simulink model "state_flow_with_system"  (R2023a)
settings: Solver=ode4  StartTime=0.0  StopTime=35  FixedStep=0.01
settings Model: Creator=Nada Tamer  LastModifiedBy=Dina
settings SolverCC: MaxConsecutiveMinStep=10  ZeroCrossAlgorithm=Adaptive
settings DebuggingCC: TimeAdjustmentMsg=warning  IgnoredZcDiagnostic=none

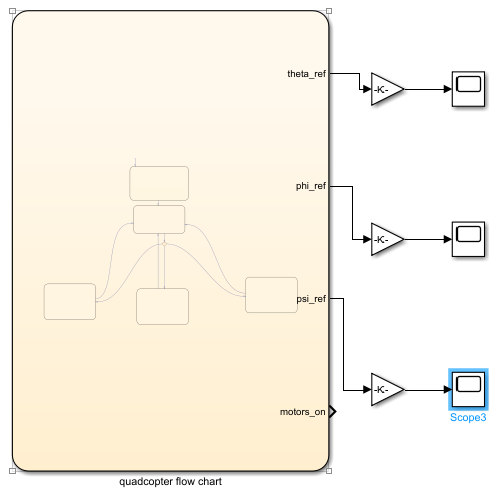
[thumbnail: Simulink's stored preview of the top-level diagram]
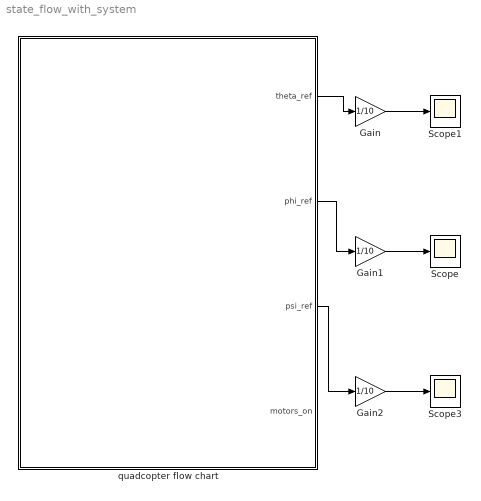
== system state_flow_with_system ==
  Gain : Gain  Gain=1/10
  Gain1 : Gain  Gain=1/10
  Gain2 : Gain  Gain=1/10
  Scope : Scope
  Scope1 : Scope
  Scope3 : Scope
  quadcopter flow chart : Stateflow chart  TreatAsAtomicUnit=on
      settings: PortSchema="{\"entries\":[{\"content\":{\"sides\":[{\"content\":{},\"type\":\"ConnectorPlacement.EquallySpacedRectSide\",\"uuid\":\"56c2e152-afcd-40b1-8237-a18b8b05acf4\"},{\"content\":{\"connectorIds\":[\"Out2\",\"Out1\",\"Out3\",\"Out4\"],\"side\":\"RIGHT\"},\"type\":\"ConnectorPlacement.EquallySpacedRectSide\",\"uuid\":\"7d307e09-fed8-4c03-9586-477b33e0d2f6\"},{\"content\":{\"side\":\"TOP\"},\"type\":\"ConnectorPlacement.EquallySpacedRectSide\",\"uuid\":\"801f95a9-7b02-4b08-94a9-99b5e12a9d94\"}]},\"type\":\"ConnectorPlacement.EquallySpacedConnector\",\"uuid\":\"5f4f8dcb-258e-4f39-8c43-71d86580ae1e\"}],\"packageUris\":[\"http://schema.mathworks.com/mf0/Connector/R2020b\"],\"version\":\"1.0\"}"
  wires:
  quadcopter flow chart/1(phi_ref) -> Gain1/1
  quadcopter flow chart/2(theta_ref) -> Gain/1
  quadcopter flow chart/3(psi_ref) -> Gain2/1
  Gain/1 -> Scope1/1
  Gain1/1 -> Scope/1
  Gain2/1 -> Scope3/1

== stateflow chart state_flow_with_system/quadcopter flow chart ==
  state Initialization
    entry:
    motor_initialization = 1;
    imu_initialization = 1;
    theta_ramp =1;
    phi_ramp =0;
    psi_ramp =0;
    motors_on = 1;
  state Zero_Stabalization_For_All
    entry:
    theta_ref = 0;
    phi_ref = 0;
    psi_ref = 0;
  state Theta_ramp
    du:
    theta_ref = theta_ref+1;
    theta_ramp =0;
    phi_ramp=1
  state Phi_ramp1
    du:
    phi_ref = phi_ref+1;
    phi_ramp =0;
    psi_ramp = 1;
  state Psi_ramp2
    du:
    psi_ref = psi_ref+1;
  (default) -> Initialization
  Initialization -> Zero_Stabalization_For_All : [motor_initialization==1&imu_initialization==1]
  Phi_ramp1 -> Zero_Stabalization_For_All : after(5,sec)
  Theta_ramp -> Zero_Stabalization_For_All : after(5,sec)
  Psi_ramp2 -> Zero_Stabalization_For_All : after(5,sec)
  Zero_Stabalization_For_All -> (junction 148) : after(5,sec)
  (junction 148) -> Phi_ramp1 [order 3] : [phi_ramp==1]
  (junction 148) -> Theta_ramp [order 2] : [theta_ramp ==1]
  (junction 148) -> Psi_ramp2 [order 1] : [psi_ramp == 1]
  data: imu_initialization local; motor_initialization local; phi_ref output; theta_ref output; psi_ref output; phi_ramp local; psi_ramp local; theta_ramp local; motors_on output
